simulink model "NonLinear_TruckTrailer"  (R2018b)
settings: Solver=VariableStepAuto  StartTime=0.0  StopTime=20  RelTol=1e-3
values from neighbouring files (symbols this model uses):
  constants = [C1 C2 C3 m1 m2 I1 I2 a1 l1 h1 b1 a2 l2 Vx]    [Dynamic_model_articulation.m]
  Vx = 20    [Dynamic_model_articulation.m]
settings Model: Creator=kevingasik  LastModifiedBy=kevingasik

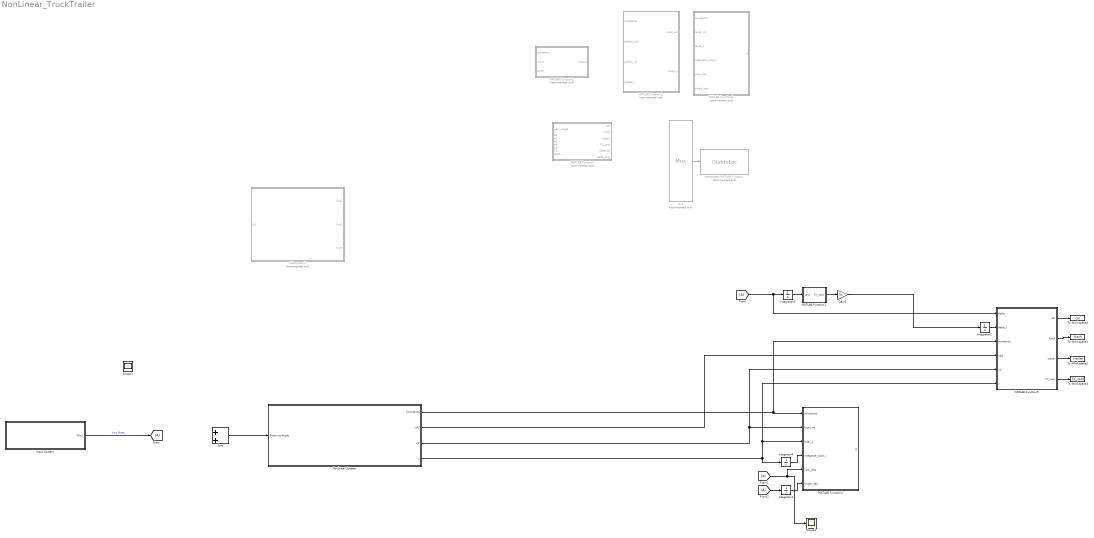
== system NonLinear_TruckTrailer ==
  Gain1 : Gain  Gain=Vx
  Input System : Subsystem
  Integrator{1..4} (4 alike) : Integrator
  Interpreted MATLAB Function : MATLABFcn  Commented=on  MATLABFcn=GlobtoLoc
  MATLAB Function : MATLAB Function  Commented=on  TreatAsAtomicUnit=on
  MATLAB Function1 : MATLAB Function  TreatAsAtomicUnit=on
  MATLAB Function2 : MATLAB Function  Commented=on  TreatAsAtomicUnit=on
  MATLAB Function3 : MATLAB Function  Commented=on  TreatAsAtomicUnit=on
  MATLAB Function4 : MATLAB Function  TreatAsAtomicUnit=on
  MATLAB Function5 : MATLAB Function  TreatAsAtomicUnit=on
  MATLAB Function6 : MATLAB Function  Commented=on  TreatAsAtomicUnit=on
  Mux : Mux  Commented=on
  Nonlinear System : Subsystem
  Scope3 : Scope
  Subsystem1 : Subsystem  Commented=on
  Sum : Sum  Inputs=|++
  To Workspace1 : ToWorkspace  VariableName=hitch  SampleTime=-1
      settings: Save2DSignal=2-D array (concatenate along first dimension)
  To Workspace2 : ToWorkspace  VariableName=trailer  SampleTime=-1
      settings: Save2DSignal=2-D array (concatenate along first dimension)
  To Workspace3 : ToWorkspace  VariableName=XY_coor  SampleTime=-1
      settings: Save2DSignal=2-D array (concatenate along first dimension)
  To Workspace4 : ToWorkspace  VariableName=car  SampleTime=-1
      settings: Save2DSignal=2-D array (concatenate along first dimension)
  Scope1 : Scope
  wires:
  Integrator3/1 -> MATLAB Function1/1(yaw)
  [A] -> MATLAB Function5/1(delta), Integrator3/1
  MATLAB Function1/1(XY_coor) -> Gain1/1
  Gain1/1 -> Integrator2/1
  Mux/1 -> Interpreted MATLAB Function/1
  Nonlinear System/4(x) -> MATLAB Function4/3(local_x), MATLAB Function5/6(x), Integrator4/1
  Nonlinear System/3(xd) -> MATLAB Function5/5(xd), MATLAB Function4/2(local_xd)
  Nonlinear System/2(xdd) -> MATLAB Function5/4(xdd)
  Nonlinear System/1(Constants) -> MATLAB Function4/1(constants), MATLAB Function5/3(constants)
  Integrator2/1 -> MATLAB Function5/2(delta_I)
  MATLAB Function5/1(car) -> To Workspace4/1
  MATLAB Function5/2(hitch) -> To Workspace1/1
  MATLAB Function5/3(trailer) -> To Workspace2/1
  MATLAB Function5/4(XY_coor) -> To Workspace3/1
  [A] -> Scope3/1, MATLAB Function4/5(yaw_des)
  [A] -> Integrator1/1
  Integrator1/1 -> MATLAB Function4/6(angle_des)
  Integrator4/1 -> MATLAB Function4/4(integrate_local_x)
  Input System/1(Out1) -> [A]  "Yaw Rate"
  Sum/1 -> Nonlinear System/1(Steering Angle)

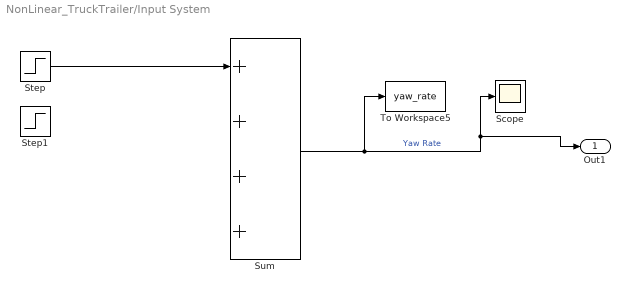
== system NonLinear_TruckTrailer/Input System ==
  Scope : Scope
  Step : Step  Time=0  After=0.5*pi/180  SampleTime=0
  Step1 : Step  After=-0.1  SampleTime=0
  Sum : Sum  Inputs=++++
  To Workspace5 : ToWorkspace  VariableName=yaw_rate  SampleTime=-1
      settings: Save2DSignal=2-D array (concatenate along first dimension)
  Out1 : Outport
  wires:
  Step/1 -> Sum/1
  Sum/1 -> To Workspace5/1, Out1/1, Scope/1  "Yaw Rate"

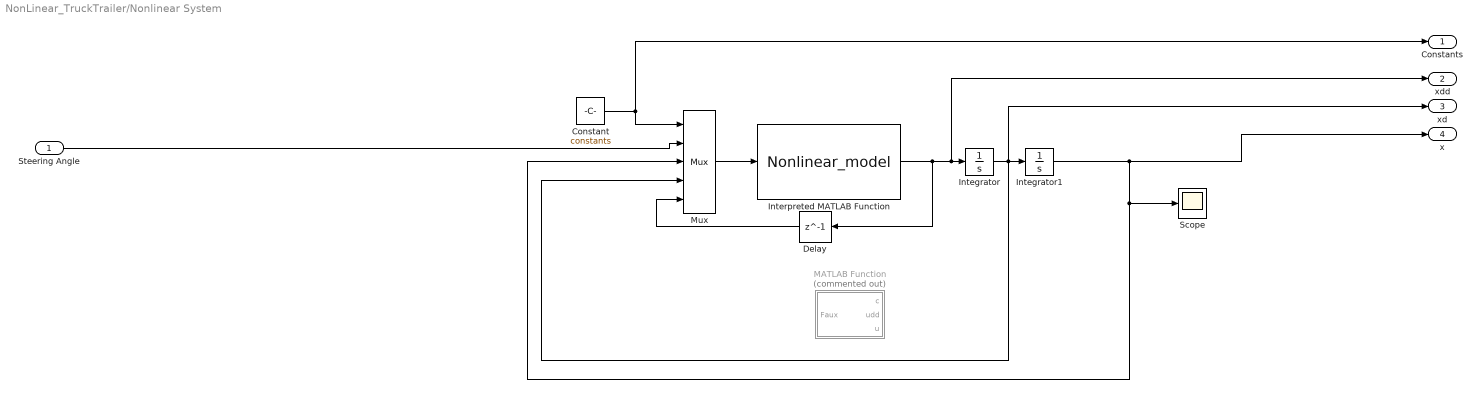
== system NonLinear_TruckTrailer/Nonlinear System ==
  Steering Angle : Inport
  Constant : Constant  Value=constants
  Delay : Delay  DelayLength=1  InitialCondition=[0 0 0 0]
  Integrator : Integrator  InitialCondition=[20 0 0 0]
  Integrator1 : Integrator  InitialCondition=[0 0 0 0]
  Interpreted MATLAB Function : MATLABFcn  MATLABFcn=Nonlinear_model
  MATLAB Function : MATLAB Function  Commented=on  TreatAsAtomicUnit=on
  Mux : Mux  Inputs=5
  Scope : Scope
  Constants : Outport
  xdd : Outport  Port=2
  xd : Outport  Port=3
  x : Outport  Port=4
  wires:
  Mux/1 -> Interpreted MATLAB Function/1
  Steering Angle/1 -> Mux/2
  Constant/1 -> Constants/1, Mux/1
  Integrator/1 -> Integrator1/1, Mux/4, xd/1
  Integrator1/1 -> Scope/1, Mux/3, x/1
  Interpreted MATLAB Function/1 -> Delay/1, xdd/1, Integrator/1
  Delay/1 -> Mux/5

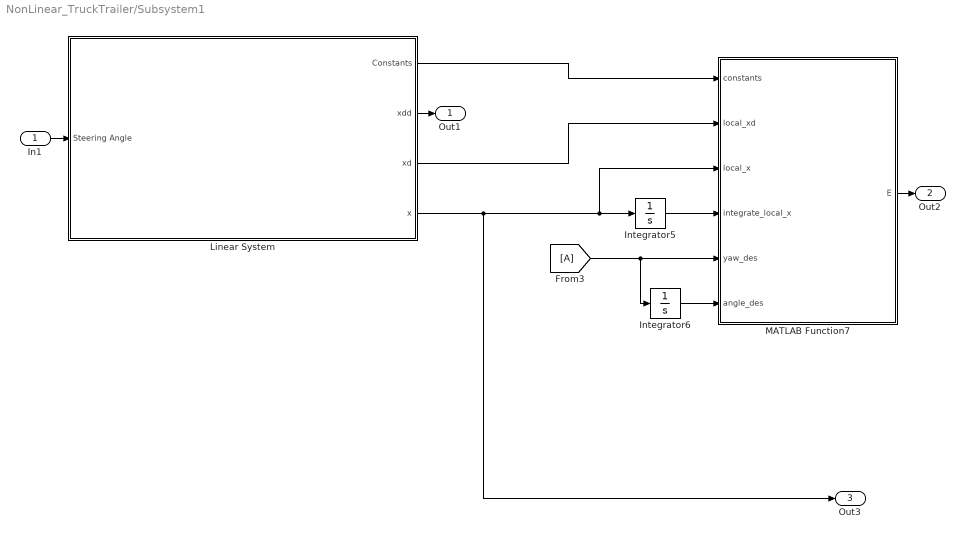
== system NonLinear_TruckTrailer/Subsystem1 ==
  In1 : Inport
  Integrator5 : Integrator
  Integrator6 : Integrator
  Linear System : Subsystem
  MATLAB Function7 : MATLAB Function  TreatAsAtomicUnit=on
  Out1 : Outport
  Out2 : Outport  Port=2
  Out3 : Outport  Port=3
  wires:
  In1/1 -> Linear System/1(Steering Angle)
  Integrator5/1 -> MATLAB Function7/4(integrate_local_x)
  Linear System/4(x) -> Out3/1, Integrator5/1, MATLAB Function7/3(local_x)
  Linear System/3(xd) -> MATLAB Function7/2(local_xd)
  Linear System/2(xdd) -> Out1/1
  [A] -> Integrator6/1, MATLAB Function7/5(yaw_des)
  MATLAB Function7/1(E) -> Out2/1
  Linear System/1(Constants) -> MATLAB Function7/1(constants)
  Integrator6/1 -> MATLAB Function7/6(angle_des)

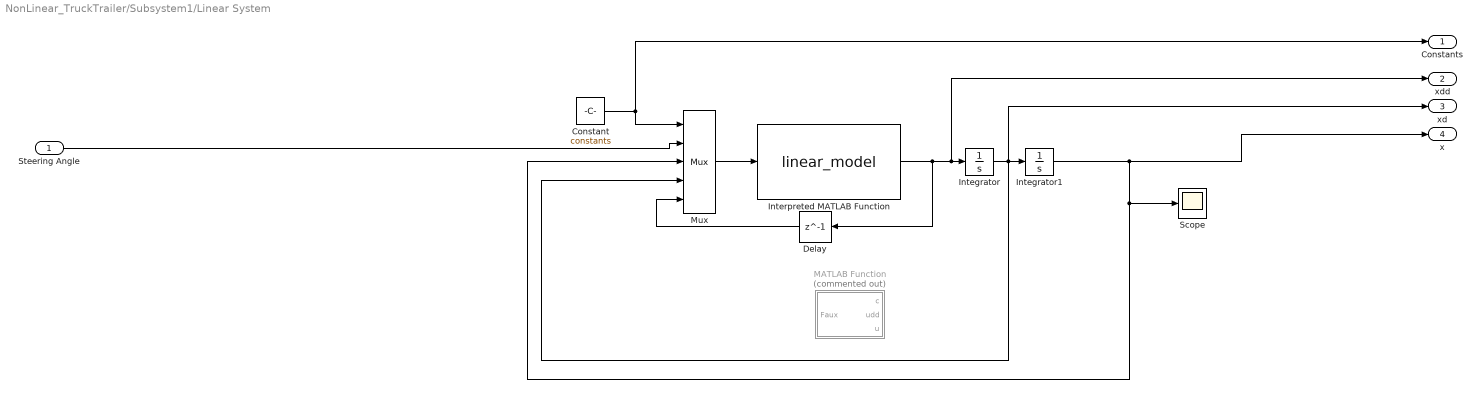
== system NonLinear_TruckTrailer/Subsystem1/Linear System ==
  Steering Angle : Inport
  Constant : Constant  Value=constants
  Delay : Delay  DelayLength=1  InitialCondition=[0 0 0 0]
  Integrator : Integrator  InitialCondition=[20 0 0 0]
  Integrator1 : Integrator  InitialCondition=[0 0 0 0]
  Interpreted MATLAB Function : MATLABFcn  MATLABFcn=linear_model
  MATLAB Function : MATLAB Function  Commented=on  TreatAsAtomicUnit=on
  Mux : Mux  Inputs=5
  Scope : Scope
  Constants : Outport
  xdd : Outport  Port=2
  xd : Outport  Port=3
  x : Outport  Port=4
  wires:
  Mux/1 -> Interpreted MATLAB Function/1
  Steering Angle/1 -> Mux/2
  Constant/1 -> Constants/1, Mux/1
  Integrator/1 -> Integrator1/1, Mux/4, xd/1
  Integrator1/1 -> Scope/1, Mux/3, x/1
  Interpreted MATLAB Function/1 -> Delay/1, xdd/1, Integrator/1
  Delay/1 -> Mux/5

== matlab function NonLinear_TruckTrailer/MATLAB Function ==
  data: yaw_angle input; r input; e1 input; car output; hitch output; trailer output; XY_coor output; e2 input; e3 input; e4 input; a2 input; h1 input; distance output; delta input; delta_ang output
function [car,hitch,trailer,XY_coor,distance,delta_ang] = fcn(yaw_angle,r,e1,e2,e3, e4, a2,h1,delta)
XY_coor = [0 0];
trailer = [0 0];
hitch = [0 0];
car = [0 0];
angle = 0;


%%Transformation matrices from local to global coordinates
Q = [-sin(yaw_angle+e2),cos(yaw_angle+e2)];
R = [-cos(yaw_angle+e2),-sin(yaw_angle+e2)];
T = [-cos(yaw_angle+e4),-sin(yaw_angle+e4)];

%% desired trajectory
X_des = r(1,1);
Y_des = r(1,2);
%X_des2 = r(1,1) - (a2+h1)*cosd(yaw_angle+e2);
%Y_des2 = r(1,2) - (a2+h1)*sind(yaw_angle+e2);
XY_coor = [X_des,Y_des];

%outputting the correct output.
car_x = r(1,1)+ e1*Q(1,1);
car_y = r(1,2)+ e1*Q(1,2);
car = [car_x,car_y];

hitch_x = r(1,1) + e1*Q(1,1) + h1*R(1,1);
hitch_y = r(1,2) + e1*Q(1,2) + h1*R(1,2);
%hitch_a = X_des2 + e3*Q(1,1) - a2*T(1,1);
%hitch_b = Y_des2 + e3*Q(1,2) - a2*T(1,2);
hitch = [hitch_x,hitch_y];


trailer_x = r(1,1)+ (e1)*Q(1,1) + h1*R(1,1) + a2*T(1,1);
trailer_y = r(1,2)+ (e1)*Q(1,2) + h1*R(1,2) + a2*T(1,2);
%trailer_x = X_des2 + e3*Q(1,1);
%trailer_y = Y_des2 + e3*Q(1,2);

distance = sqrt((abs(hitch_x-trailer_x))^2 + abs(hitch_y-trailer_y)^2);
delta_ang = delta + e2 + yaw_angle; 
trailer = [trailer_x,trailer_y];

== matlab function NonLinear_TruckTrailer/MATLAB Function1 ==
  data: yaw input; XY_coor output
function XY_coor  = fcn(yaw)

XY_coor = [cos(yaw),sin(yaw)];

== matlab function NonLinear_TruckTrailer/MATLAB Function2 ==
  data: output output; constants input; input input; LOTS input
function output  = fcn(constants,input,LOTS)
coder.extrinsic('NonLinearFunction');
output = [0;0;0;0];

[output] = NonLinearFunction(constants,input,LOTS);

== matlab function NonLinear_TruckTrailer/MATLAB Function3 ==
  data: constants input; global_xdd input; global_xd input; global_x input; local_xd output; local_x output
function [local_xd,local_x] = fcn(constants,global_xdd,global_xd, global_x)
%% this function takes the global coordinates from the nonlinear system and
%% converts it to local coordinates to be controlled
local_x = [0 0 0 0];
local_xd = [0 0 0 0];

constants = constants';

u = constants(14);
global_x = global_x';
global_xd = global_xd';
global_xdd = global_xdd';

x = global_x(1);
y1 = global_x(2);
yaw_angle = global_x(3);
theta = global_x(4); 

xd = global_xd(1); 
y1d = global_xd(2); 
yaw_d = global_xd(3);
theta_d = global_xd(4);

xdd = global_xdd(1);
y1dd = global_xdd(2);
yaw_dd = global_xdd(3);
theta_dd = global_xdd(4);

v1 = y1d - u*yaw_angle;
psi_d = yaw_d;
phi_d = theta_d - yaw_d;
phi = theta - yaw_angle;
local_x = [v1 psi_d phi_d phi]; 


v1d = y1dd - u*yaw_d;
psi_dd = yaw_dd;
phi_dd = theta_dd-yaw_dd;
phi_d = theta_d - yaw_d;
local_xd = [v1d psi_dd phi_dd phi_d];

== matlab function NonLinear_TruckTrailer/MATLAB Function4 ==
  data: constants input; local_xd input; local_x input; integrate_local_x input; E output; yaw_des input; angle_des input
function E  = fcn(constants,local_xd,local_x,integrate_local_x,yaw_des,angle_des)
%% this function takes the local coordinates and converts them into error coordinates
%% to be controlled
E = [0;0;0;0];

Vx = constants(14);
a2 = constants(12);

yaw = integrate_local_x(2);

v1 = local_x(2);
psi_d = local_x(3);

v1d = local_xd(2);
psi_dd = local_xd(3);



e1d = v1d + Vx*(yaw-angle_des);
e2d = yaw - angle_des;

e1dd = v1d + Vx*(psi_d-yaw_des);
e2dd = psi_d - yaw_des;



E = [e1d;e1dd;e2d;e2dd]

== matlab function NonLinear_TruckTrailer/MATLAB Function5 ==
  data: delta input; delta_I input; constants input; xdd input; xd input; x input; car output; hitch output; trailer output; XY_coor output
function [car,hitch,trailer,XY_coor] = fcn(delta,delta_I,constants,xdd,xd,x)
XY_coor = [0 0];
trailer = [0 0];
hitch = [0 0];
car = [0 0];
angle = 0;


C1 = constants(1);
C2 = constants(2);
C3 = constants(3);
m1 = constants(4);
m2 = constants(5);
I1 = constants(6);
I2 = constants(7);
a1 = constants(8);
l1 = constants(9);
h1 = constants(10);
b1 = constants(11);
a2 = constants(12);
l2 = constants(13);
u = constants(14);

l2 = b1; 
b1 = a2;

car_x = x(1);
car_y = x(2);

%hitch_x = x(1) - l2*cos(x(3));
%hitch_y = x(2) - l2*sin(x(3));
  
%trailer_x = x(1) - l2*cos(x(3)) - b1*cos(x(4));
%trailer_y = x(2) - l2*sin(x(3)) - b1*cos(x(4));


XY_coor = delta_I;
car = [car_x, car_y];
%hitch = [hitch_x,hitch_y];
%trailer = [trailer_x, trailer_y];

== matlab function NonLinear_TruckTrailer/Nonlinear System/MATLAB Function ==
  data: c input; udd input; u input; Faux output
function Faux = fcn(c,udd,u)

m1 = c;
xdd = udd(1) ;
ydd = udd(2) ;


beta = u(3) ;
theta = u(4);
Faux_x = m1*x_dd - Fyf1*cos(beta+delta) - Fyr1*cos(beta);
Faux_y = m1*y_dd - Fyf1*sin(beta+delta) - Fyr1*sin(beta);

Faux = sqrt(Faux_x^2 + Faux_y^2);

== matlab function NonLinear_TruckTrailer/MATLAB Function6 ==
  data: constants input; local_xd input; local_x input; integrate_local_x input; E output; yaw_des input; angle_des input
function E  = fcn(constants,local_xd,local_x,integrate_local_x,yaw_des,angle_des)
%% this function takes the local coordinates and converts them into error coordinates
%% to be controlled
E = [0;0;0;0;0;0;0;0];


Vx = constants(14);
a2 = constants(12);

yaw = integrate_local_x(2);

v1 = local_x(1);
psi_d = local_x(2);
phi_d = local_x(3);
phi = local_x(4);

v1d = local_xd(1);
psi_dd = local_xd(2);
phi_dd = local_xd(3);
phi_d = local_xd(4);


e1d = v1d + Vx*(yaw-angle_des);
e2d = yaw - angle_des;
e3d = v1d + phi_d*a2 + Vx*(phi + yaw - angle_des);
e4d = phi_d + psi_d - yaw_des;

e1dd = v1d + Vx*(psi_d-yaw_des);
e2dd = psi_d - yaw_des;
e3dd = v1d + phi_dd*a2 + Vx*(phi_d+psi_d-yaw_des);
e4dd = phi_d + psi_dd;


E = [e1d;e1dd;e2d;e2dd;e3d;e3dd;e4d;e4dd];

== matlab function NonLinear_TruckTrailer/Subsystem1/Linear System/MATLAB Function ==
  data: c input; udd input; u input; Faux output
function Faux = fcn(c,udd,u)

m1 = c;
xdd = udd(1) ;
ydd = udd(2) ;


beta = u(3) ;
theta = u(4);
Faux_x = m1*x_dd - Fyf1*cos(beta+delta) - Fyr1*cos(beta);
Faux_y = m1*y_dd - Fyf1*sin(beta+delta) - Fyr1*sin(beta);

Faux = sqrt(Faux_x^2 + Faux_y^2);

== matlab function NonLinear_TruckTrailer/Subsystem1/MATLAB Function7 ==
  data: constants input; local_xd input; local_x input; integrate_local_x input; E output; yaw_des input; angle_des input
function E  = fcn(constants,local_xd,local_x,integrate_local_x,yaw_des,angle_des)
%% this function takes the local coordinates and converts them into error coordinates
%% to be controlled
E = [0;0;0;0];

Vx = constants(14);
a2 = constants(12);

yaw = integrate_local_x(2);

v1 = local_x(2);
psi_d = local_x(3);

v1d = local_xd(2);
psi_dd = local_xd(3);



e1d = v1d + Vx*(yaw-angle_des);
e2d = yaw - angle_des;

e1dd = v1d + Vx*(psi_d-yaw_des);
e2dd = psi_d - yaw_des;



E2 = [e1d;e1dd;e2d;e2dd]
